simulink model "PositionPI_limberoGrieel_leg_control_DH"  (R2022a)
settings: Solver=ode45  StartTime=0.0  StopTime=8.00  RelTol=1e-3
values from neighbouring files (symbols this model uses):
  a = annotation('textbox',dim,'String',str,'FontSize', 20, 'FitBoxToText','on', 'Interpreter', 'tex')    [Experiment_Plot_csv.m]    (also in GRIEEL_transform.m; Gazebo_Plot_csv.m; Grasshopper_Manipulability.m = [a_1; a_2; a_3]; Hexapod_Manipulability_Develop_limits.m = [0, a2, a3])
  a_contact = [a1_contact, a2_contact, 0, a4_contact, a5_contact, a6_contact, 0]    [LimberoGrieel_Leg_DH_Modeling_Control.m]    (also in NewLimbManipulabilityTest.m = [a2, 0, 0]; NewRobot_Manipulability_Test.m = [a2, 0, 0]; limberoGrieel_leg_DH.m; limbero_grieel_dh.m)
  alpha = [alpha; alpha; alpha]    [Grasshopper_Manipulability.m]    (also in Hexapod_Manipulability_Develop_limits.m = [-pi/2, 0, 0]; LimberoGrieel_Leg_DH_Modeling_Control.m = [-pi/2,0,0,-pi/2,pi/2, -pi/2, 0]; NewLimbManipulabilityTest.m = [-pi/2, 0, 0]; NewRobot_Manipulability_Develop.m = [-pi/2, 0, 0])
  alpha_contact = [-pi/2, pi/2, -pi/2, 0, 0, -pi/2, 0]    [LimberoGrieel_Leg_DH_Modeling_Control.m]    (also in NewLimbManipulabilityTest.m = [0, pi/2, 0]; NewRobot_Manipulability_Test.m = [0, pi/2, 0]; limberoGrieel_leg_DH.m; limbero_grieel_dh.m)
  d = [d; d; d; d]    [Grasshopper_Manipulability.m]    (also in Hexapod_Manipulability_Develop_limits.m = [0, 0, 0]; LimberoGrieel_Leg_DH_Modeling_Control.m = [0,0,0,0,d5,0,d7]; NewLimbManipulabilityTest.m = [d1, 0, 0]; NewRobot_Manipulability_Develop.m = [d1, 0, 0])
  d_contact = [0, 0, d3_contact, 0, 0, 0, d7_contact]    [LimberoGrieel_Leg_DH_Modeling_Control.m]    (also in NewLimbManipulabilityTest.m = [0, 0, -d1]; NewRobot_Manipulability_Test.m = [0, 0, -d1]; limberoGrieel_leg_DH.m; limbero_grieel_dh.m)
  kpp = w_cp    (= 10)    [LimberoGrieel_Leg_DH_Modeling_Control.m]    (also in limberoGrieel_leg_DH.m = 20; limbero_controller.mat; limbero_grieel_dh.m = 20)
  kpv = zeros(1,7)    [LimberoGrieel_Leg_DH_Modeling_Control.m]    (also in limberoGrieel_leg_DH.m; limbero_controller.mat = [361.431320062 321.270503754 225.035980044 266.544083168 222; limbero_grieel_dh.m)
  L = 0.25    [Experiment_Plot_csv.m]    (also in Gazebo_Plot_csv.m; Grasshopper_Manipulability.m = 0.5; Hexapod_Manipulability_Develop_limits.m = 0.45; LimberoGrieel_Leg_DH_Modeling_Control.m = 30)
  masses = zeros(N_link,1)    [LimberoGrieel_Leg_DH_Modeling_Control.m]    (also in limberoGrieel_leg_DH.m; limbero_controller.mat = [0.09109 0.12821 0.061841 0.081999 0.110299813858 0.13265995; limbero_grieel_dh.m)
  masses_contact = zeros(N_link,1)    [LimberoGrieel_Leg_DH_Modeling_Control.m]    (also in limberoGrieel_leg_DH.m; limbero_grieel_dh.m)
  offset = [offset; offset; offset]    [Grasshopper_Manipulability.m]    (also in Hexapod_Manipulability_Develop_limits.m = [0, 0, 0]; LimberoGrieel_Leg_DH_Modeling_Control.m = zeros(N_link,1); NewLimbManipulabilityTest.m = [0, 0, 0]; NewRobot_Manipulability_Develop.m = [0, 0, 0])
  offset_contact = zeros(N_link,1)    [LimberoGrieel_Leg_DH_Modeling_Control.m]    (also in NewLimbManipulabilityTest.m = [0, 0, pi]; NewRobot_Manipulability_Test.m = [0, 0, pi]; limberoGrieel_leg_DH.m; limbero_grieel_dh.m)
  q_dotdot = zeros(1,7)    [limberoGrieel_leg_DH.m]    (also in limbero_grieel_dh.m)
  qz = zeros(1,limbero.n)    [LimberoGrieel_Leg_DH_Modeling_Control.m]    (also in NewLimbManipulabilityTest.m = zeros(1,Limb_swing.n); NewRobot_Manipulability_Test.m = zeros(1,Limb_swing.n); limberoGrieel_leg_DH.m; limberoGrieel_model_DH.m)
  r_cm = zeros(N_link,3)    [LimberoGrieel_Leg_DH_Modeling_Control.m]    (also in limberoGrieel_leg_DH.m; limbero_controller.mat = [-0.015062 -0.09917 -0.09702 -9.53000073933e-12 -0.012686054; limbero_grieel_dh.m)
  r_cm_contact = zeros(N_link,3)    [LimberoGrieel_Leg_DH_Modeling_Control.m]    (also in limberoGrieel_leg_DH.m; limbero_grieel_dh.m)
  t0 = (ROBOT(i).base.R)'*T_base_in(1:3,1:3)*t_ee(1:3,4)    [LimberoGrieel_Robot_Manipulaibilty_Test2.m]    (also in NewLimbManipulabilityTest.m; NewRobot_Manipulability_Test.m; Robot_DH_kin.m; limberoGrieel_leg_DH.m = 0.5)
  t_acc = zeros(1,7)    [limberoGrieel_leg_DH.m]    (also in limbero_grieel_dh.m)
  T_lpf = 1/(w_lpf*2*pi)    (= 0.0106103295395)    [LimberoGrieel_Leg_DH_Modeling_Control.m]    (also in limberoGrieel_leg_DH.m; limbero_controller.mat; limbero_grieel_dh.m)
  t_tot = 2.5    [limberoGrieel_leg_DH.m]    (also in limbero_grieel_dh.m)
  T_vel = 1/(w_vel*2*pi)    (= 0.00318309886184)    [LimberoGrieel_Leg_DH_Modeling_Control.m]    (also in limberoGrieel_leg_DH.m; limbero_controller.mat; limbero_grieel_dh.m)
  Tc = Tiv*0.1    (= 0.0666666666667)    [LimberoGrieel_Leg_DH_Modeling_Control.m]    (also in limberoGrieel_leg_DH.m = 0.0333333333333; limbero_controller.mat; limbero_grieel_dh.m = 0.0333333333333)
  Tiv = Tiv*10    (= 0.666666666667)    [LimberoGrieel_Leg_DH_Modeling_Control.m]    (also in limberoGrieel_leg_DH.m = 0.333333333333; limbero_controller.mat; limbero_grieel_dh.m = 0.333333333333)
libraries: roblocks x6
(part 2 of 2)

== system PositionPI_limberoGrieel_leg_control_DH/Joint_Traj Generator/Subsystem1 ==
  Add : Sum  Inputs=++++
  Add1 : Sum
  Constant : Constant  Value=qz(3)
  Integrator : Integrator
  Integrator1 : Integrator
  Scope : Scope
  Scope1 : Scope
  Scope2 : Scope
  Step : Step  Time=t0  After=q_dotdot(3)  SampleTime=0
  Step1 : Step  Time=t0+t_acc(3)  After=-q_dotdot(3)  SampleTime=0
  Step2 : Step  Time=t0+t_tot-t_acc(3)  After=-q_dotdot(3)  SampleTime=0
  Step3 : Step  Time=t0+t_tot  After=q_dotdot(3)  SampleTime=0
  C2F : Outport
  wires:
  Add1/1 -> Scope/1, C2F/1
  Constant/1 -> Add1/1
  Integrator/1 -> Integrator1/1, Scope1/1
  Step/1 -> Add/1
  Step2/1 -> Add/3
  Step1/1 -> Add/2
  Integrator1/1 -> Add1/2
  Add/1 -> Integrator/1, Scope2/1
  Step3/1 -> Add/4

== system PositionPI_limberoGrieel_leg_control_DH/Joint_Traj Generator1/Subsystem ==
  Add : Sum  Inputs=++++
  Add1 : Sum
  Constant : Constant  Value=qz(2)
  Integrator : Integrator
  Integrator1 : Integrator
  Scope : Scope
  Scope1 : Scope
  Scope2 : Scope
  Step : Step  Time=t0  After=q_dotdot(2)  SampleTime=0
  Step1 : Step  Time=t0+t_acc(2)  After=-q_dotdot(2)  SampleTime=0
  Step2 : Step  Time=t0+t_tot-t_acc(2)  After=-q_dotdot(2)  SampleTime=0
  Step3 : Step  Time=t0+t_tot  After=q_dotdot(2)  SampleTime=0
  B2C : Outport
  wires:
  Step3/1 -> Add/4
  Add/1 -> Scope2/1, Integrator/1
  Integrator1/1 -> Add1/2
  Step1/1 -> Add/2
  Step2/1 -> Add/3
  Step/1 -> Add/1
  Integrator/1 -> Scope1/1, Integrator1/1
  Constant/1 -> Add1/1
  Add1/1 -> B2C/1, Scope/1

== system PositionPI_limberoGrieel_leg_control_DH/Joint_Traj Generator1/Subsystem1 ==
  Add : Sum  Inputs=++++
  Add1 : Sum
  Constant : Constant  Value=qz(3)
  Integrator : Integrator
  Integrator1 : Integrator
  Scope : Scope
  Scope1 : Scope
  Scope2 : Scope
  Step : Step  Time=t0  After=q_dotdot(3)  SampleTime=0
  Step1 : Step  Time=t0+t_acc(3)  After=-q_dotdot(3)  SampleTime=0
  Step2 : Step  Time=t0+t_tot-t_acc(3)  After=-q_dotdot(3)  SampleTime=0
  Step3 : Step  Time=t0+t_tot  After=q_dotdot(3)  SampleTime=0
  C2F : Outport
  wires:
  Add1/1 -> Scope/1, C2F/1
  Constant/1 -> Add1/1
  Integrator/1 -> Integrator1/1, Scope1/1
  Step/1 -> Add/1
  Step2/1 -> Add/3
  Step1/1 -> Add/2
  Integrator1/1 -> Add1/2
  Add/1 -> Integrator/1, Scope2/1
  Step3/1 -> Add/4

== matlab function PositionPI_limberoGrieel_leg_control_DH/MATLAB Function1 ==
  data: q input; g output; d parameter; a parameter; alpha parameter; offset parameter; r_cm parameter; masses parameter
function g = fcn(q, d, a, alpha, offset, r_cm, masses)
g = Gravity_compensation(a,d,alpha,offset, r_cm, masses, q, 0);

== matlab function PositionPI_limberoGrieel_leg_control_DH/MATLAB Function ==
  data: q input; g output; d parameter; a parameter; alpha parameter; offset parameter; r_cm parameter; masses parameter
function g = fcn(q, d, a, alpha, offset, r_cm, masses)
g = Gravity_compensation(a,d,alpha,offset, r_cm, masses, q, 0);

== matlab function PositionPI_limberoGrieel_leg_control_DH/MATLAB Function2 ==
  data: q input; g output; d parameter; a parameter; alpha parameter; offset parameter; r_cm parameter; masses parameter
function g = fcn(q, d, a, alpha, offset, r_cm, masses)
g = Gravity_compensation(a,d,alpha,offset, r_cm, masses, q, 0);

== matlab function PositionPI_limberoGrieel_leg_control_DH/MATLAB Function3 ==
  data: q input; g output; d_contact parameter; a_contact parameter; alpha_contact parameter; offset_contact parameter; r_cm_contact parameter; masses_contact parameter
function g = fcn(q, d_contact, a_contact, alpha_contact, offset_contact, r_cm_contact, masses_contact)
g = Gravity_compensation(a_contact,d_contact,alpha_contact,offset_contact, r_cm_contact, masses_contact, q, 1);
